simulink model "A_ZH_Z2"  (R2025a)
settings: Solver=VariableStepAuto  StartTime=0.0  StopTime=10  RelTol=1e-3
settings Model: Creator=Szalay  LastModifiedBy=Szalay

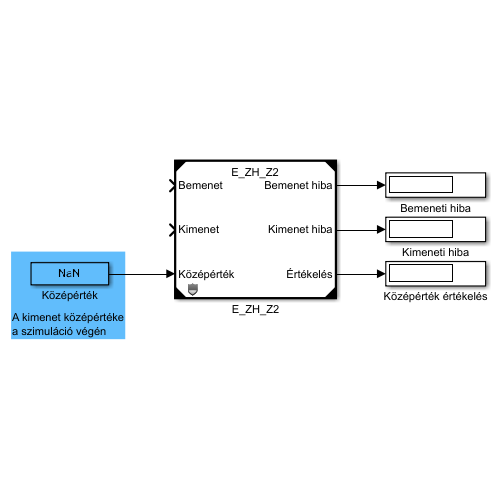
[thumbnail: Simulink's stored preview of the top-level diagram]
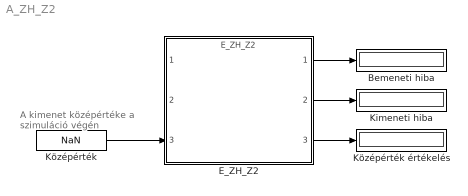
== system A_ZH_Z2 ==
  note: A kimenet középértéke
      | a szimuláció végén
  Bemeneti hiba : Display
  E_ZH_Z2 : ModelReference  ModelNameDialog=E_ZH_Z2.slxp  ModelReferenceVersion=1.14  CopyOfModelProtected=on
  Kimeneti hiba : Display
  Középérték : Constant  Value=NaN
  Középérték értékelés : Display
  wires:
  E_ZH_Z2/1 -> Bemeneti hiba/1
  E_ZH_Z2/2 -> Kimeneti hiba/1
  E_ZH_Z2/3 -> Középérték értékelés/1
  Középérték/1 -> E_ZH_Z2/3
